simulink model "SimulinkLigaDesligaSensoresVies2"  (R2013b)
settings: Solver=ode3  StartTime=0.0  StopTime=20  RelTol=1e-3
values from neighbouring files (symbols this model uses):
  Ad = [1 T ... (first row only)    [inicializaComViesAccVel.m]
  Ad_K = [1 T  0 ... (first row only)    [inicializaComViesAccVel.m]
  Bd = [T^2/2 ... (first row only)    [inicializaComViesAccVel.m]
  Bd_K = [T^2/2 ... (first row only)    [inicializaComViesAccVel.m]
  Bd_n = [T^2/2  0 ... (first row only)    [inicializaComViesAccVel.m]
  C = [1 0 ... (first row only)    [inicializaComViesAccVel.m]
  C_K = [1 0 0 ... (first row only)    [inicializaComViesAccVel.m]
  C_K1 = [1 0 0 ... (first row only)    [inicializaComViesAccVel.m]
settings Model: Creator=ThiagoCordeiro  LastModifiedBy=ThiagoFelippe

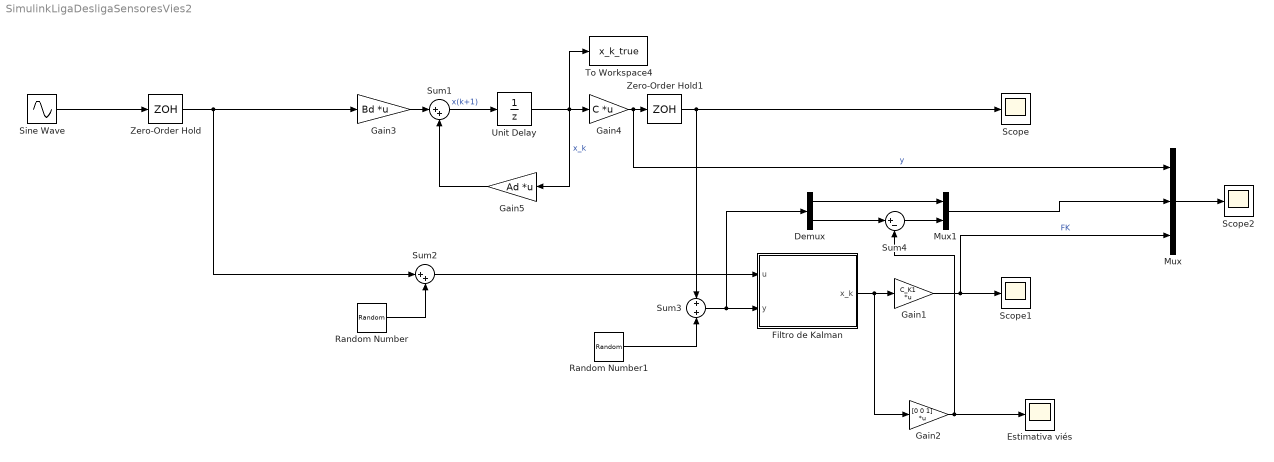
== system SimulinkLigaDesligaSensoresVies2 ==
  Demux : Demux  Outputs=2
  Estimativa viés : Scope
      settings: SaveName=ScopeData3
  Filtro de Kalman : Subsystem
  Gain1 : Gain  Gain=C_K1  Multiplication=Matrix(K*u)
  Gain2 : Gain  Gain=[0 0 1]  Multiplication=Matrix(K*u)
  Gain3 : Gain  Gain=Bd  Multiplication=Matrix(K*u)
  Gain4 : Gain  Gain=C  Multiplication=Matrix(K*u)
  Gain5 : Gain  Gain=Ad  Multiplication=Matrix(K*u)
  Mux : Mux  Inputs=3
  Mux1 : Mux  Inputs=2
  Random Number : RandomNumber  Seed=round(rand(1)*(2^32-1))  SampleTime=0.01
  Random Number1 : RandomNumber  Mean=[0; 10]  Variance=[1, 1]  Seed=round(rand(2,1)*(2^32-1))  SampleTime=0.01
  Scope : Scope
  Scope1 : Scope
  Scope2 : Scope
      settings: ShowLegends=on  SaveName=ScopeData2
  Sine Wave : Sin  Phase=pi/2  SampleTime=0
  Sum1 : Sum  Inputs=|++
  Sum2 : Sum  Inputs=|++
  Sum3 : Sum  Inputs=+|+
  Sum4 : Sum  Inputs=|+-
  To Workspace4 : ToWorkspace  VariableName=x_k_true  SampleTime=-1  SaveFormat=Timeseries
  Unit Delay : UnitDelay  InitialCondition=[0;0]  SampleTime=-1
  Zero-Order Hold : ZeroOrderHold  SampleTime=0.01
  Zero-Order Hold1 : ZeroOrderHold  SampleTime=0.01
  wires:
  Gain3/1 -> Sum1/1
  Sum1/1 -> Unit Delay/1  "x(k+1)"
  Unit Delay/1 -> To Workspace4/1, Gain4/1, Gain5/1  "x_k"
  Gain5/1 -> Sum1/2
  Filtro de Kalman/1(x_k) -> Gain2/1, Gain1/1
  Gain1/1 -> Mux/3, Scope1/1  "FK"
  Mux/1 -> Scope2/1
  Zero-Order Hold/1 -> Sum2/1, Gain3/1
  Sum2/1 -> Filtro de Kalman/1(u)
  Random Number/1 -> Sum2/2
  Sum3/1 -> Demux/1, Filtro de Kalman/2(y)
  Random Number1/1 -> Sum3/2
  Zero-Order Hold1/1 -> Scope/1, Sum3/1
  Gain4/1 -> Mux/1, Zero-Order Hold1/1  "y"
  Sine Wave/1 -> Zero-Order Hold/1
  Gain2/1 -> Estimativa viés/1, Sum4/2
  Mux1/1 -> Mux/2
  Demux/1 -> Mux1/1
  Demux/2 -> Sum4/1
  Sum4/1 -> Mux1/2

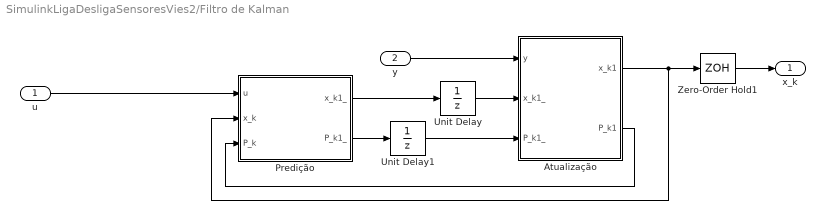
== system SimulinkLigaDesligaSensoresVies2/Filtro de Kalman ==
  u : Inport
  y : Inport  Port=2
  Atualização : Subsystem
  Predição : Subsystem
  Unit Delay : UnitDelay  InitialCondition=[5;-3;0]*0  SampleTime=0.01
  Unit Delay1 : UnitDelay  InitialCondition=[5 0 0; 0 5 0; 0 0 100];  SampleTime=0.01
  Zero-Order Hold1 : ZeroOrderHold  SampleTime=0.01
  x_k : Outport
  wires:
  u/1 -> Predição/1(u)
  y/1 -> Atualização/1(y)
  Atualização/1(x_k1) -> Predição/2(x_k), Zero-Order Hold1/1
  Atualização/2(P_k1) -> Predição/3(P_k)
  Zero-Order Hold1/1 -> x_k/1
  Predição/2(P_k1_) -> Unit Delay1/1
  Unit Delay1/1 -> Atualização/3(P_k1_)
  Unit Delay/1 -> Atualização/2(x_k1_)
  Predição/1(x_k1_) -> Unit Delay/1

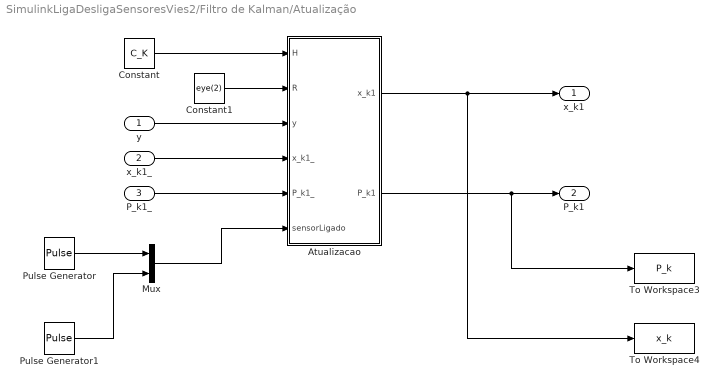
== system SimulinkLigaDesligaSensoresVies2/Filtro de Kalman/Atualização ==
  y : Inport
  x_k1_ : Inport  Port=2
  P_k1_ : Inport  Port=3
  Atualizacao : MATLAB Function  TreatAsAtomicUnit=on  SystemSampleTime=0.01
  Constant : Constant  Value=C_K  VectorParams1D=off
  Constant1 : Constant  Value=eye(2)
  Mux : Mux  Inputs=2
  Pulse Generator : DiscretePulseGenerator  Period=3  SampleTime=0.01
  Pulse Generator1 : DiscretePulseGenerator  Period=5  SampleTime=0.01
  To Workspace3 : ToWorkspace  VariableName=P_k  SampleTime=-1  SaveFormat=Timeseries
  To Workspace4 : ToWorkspace  VariableName=x_k  SampleTime=-1  SaveFormat=Timeseries
  x_k1 : Outport
  P_k1 : Outport  Port=2
  wires:
  y/1 -> Atualizacao/3(y)
  x_k1_/1 -> Atualizacao/4(x_k1_)
  P_k1_/1 -> Atualizacao/5(P_k1_)
  Atualizacao/1(x_k1) -> To Workspace4/1, x_k1/1
  Atualizacao/2(P_k1) -> To Workspace3/1, P_k1/1
  Constant/1 -> Atualizacao/1(H)
  Constant1/1 -> Atualizacao/2(R)
  Pulse Generator/1 -> Mux/1
  Pulse Generator1/1 -> Mux/2
  Mux/1 -> Atualizacao/6(sensorLigado)

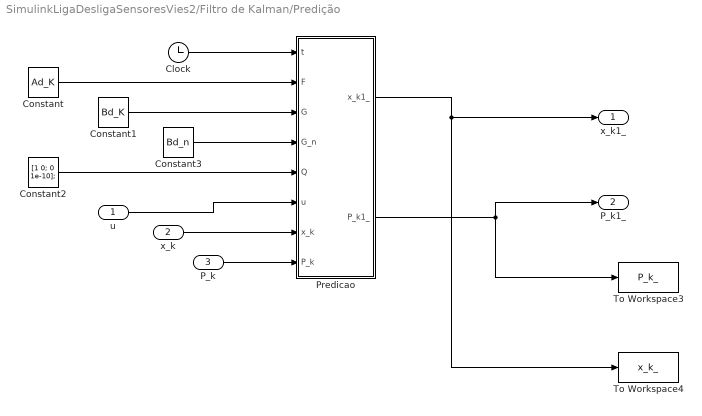
== system SimulinkLigaDesligaSensoresVies2/Filtro de Kalman/Predição ==
  u : Inport
  x_k : Inport  Port=2
  P_k : Inport  Port=3
  Clock : Clock
  Constant : Constant  Value=Ad_K
  Constant1 : Constant  Value=Bd_K  VectorParams1D=off
  Constant2 : Constant  Value=[1 0; 0 1e-10];
  Constant3 : Constant  Value=Bd_n  VectorParams1D=off
  Predicao : MATLAB Function  TreatAsAtomicUnit=on  SystemSampleTime=0.01
  To Workspace3 : ToWorkspace  VariableName=P_k_  SampleTime=-1  SaveFormat=Timeseries
  To Workspace4 : ToWorkspace  VariableName=x_k_  SampleTime=-1  SaveFormat=Timeseries
  x_k1_ : Outport
  P_k1_ : Outport  Port=2
  wires:
  u/1 -> Predicao/6(u)
  x_k/1 -> Predicao/7(x_k)
  P_k/1 -> Predicao/8(P_k)
  Constant/1 -> Predicao/2(F)
  Constant1/1 -> Predicao/3(G)
  Constant2/1 -> Predicao/5(Q)
  Predicao/1(x_k1_) -> To Workspace4/1, x_k1_/1
  Predicao/2(P_k1_) -> P_k1_/1, To Workspace3/1
  Clock/1 -> Predicao/1(t)
  Constant3/1 -> Predicao/4(G_n)

== matlab function SimulinkLigaDesligaSensoresVies2/Filtro de Kalman/Atualização/Atualizacao ==
  data: H input; R input; y input; x_k1_ input; P_k1_ input; x_k1 output; P_k1 output; sensorLigado input
function [x_k1, P_k1] = fcn(H, R, y, x_k1_, P_k1_, sensorLigado)
%#codegen

if (sensorLigado(1) == 0) && (sensorLigado(2) == 0)
    x_k1 = x_k1_; 
    P_k1 = P_k1_;
else
    faixaVal = sensorLigado == 1;
    H_ = H(faixaVal,:);
    R_ = R(faixaVal,faixaVal);
    y_ = y(faixaVal);
    [x_k1, P_k1] = pred(H_, R_, y_, x_k1_, P_k1_);
end
end

function [x_k1, P_k1] = pred(H, R, y, x_k1_, P_k1_)
% Trecho abaixo nao depende nem do estado estimado, nem da medida obtida,
% entao pode ser calculado offline e armazenado em tabela
S = H * P_k1_ * H' + R;
Pxy = P_k1_ * H';
K_k  =  Pxy / S;
KH = K_k*H;
I = eye(size(KH));
I_KH = I - KH;
P_k1 = I_KH * P_k1_ * I_KH' + K_k * R * K_k';
% --- fim do trecho que pode ser calculado offline

y_hat = H * x_k1_;
y_tilde = y - y_hat;
x_k1 = x_k1_ + K_k * y_tilde;

end

== matlab function SimulinkLigaDesligaSensoresVies2/Filtro de Kalman/Predição/Predicao ==
  data: t input; F input; G input; G_n input; Q input; u input; x_k1_ output; x_k input; P_k input; P_k1_ output
function [x_k1_,P_k1_] = fcn(t, F, G, G_n, Q, u, x_k, P_k)
%#codegen
if t >= 0
    x_k1_ = F*x_k + G*u;
    P_k1_ = F*P_k*F' + G_n*Q*G_n';
else
    x_k1_ = x_k;
    P_k1_ = P_k;
end
